simulink model "verify_Thermostat_Proportional_mdl"  (R2016b)
settings: Solver=ode45  StartTime=0.0  StopTime=100  MaxStep=1  RelTol=1e-3  EnableMultiTasking=on
libraries: simulink x1, carnot x1
settings Model: Creator=drhf  LastModifiedBy=drhf
settings DataIOCC: SaveFormat=Array  SignalLoggingSaveFormat=ModelDataLogs
settings OptimizationCC: ExpressionDepthLimit=2147483647  LifeSpan=inf
settings DebuggingCC: UnderspecifiedInitializationDetection=Classic  MergeDetectMultiDrivingBlocksExec=none  SolverPrmCheckMsg=warning  FcnCallInpInsideContextMsg=warning  StateNameClashWarn=warning  SFUnexpectedBacktrackingDiag=warning  SFNoUnconditionalDefaultTransitionDiag=warning  SFExecutionAtInitializationDiag=none
settings HardwareCC: ProdBitPerPointer=32  ProdBitPerSizeT=32  ProdBitPerPtrDiffT=32  ProdLargestAtomicFloat=None  ProdIntDivRoundTo=Undefined  ProdEndianess=Unspecified  ProdWordSize=32  ProdHWDeviceType=32-bit Generic
settings ModelReferenceCC: PropagateSignalLabelsOutOfModel=off
settings GRTTargetCC: TargetLangStandard=C89/C90 (ANSI)  GeneratePreprocessorConditionals=Disable all  CombineOutputUpdateFcns=off  GRTInterface=on
settings ConfigComp: CovMetricSettings=dw  CovHtmlReporting=on  CovSaveCumulativeToWorkspaceVar=on  CovSaveSingleToWorkspaceVar=on  CovExternalEMLEnable=off

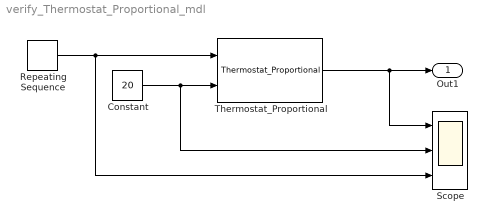
== system verify_Thermostat_Proportional_mdl ==
  Constant : Constant  Value=20
  Repeating Sequence : simulink/Sources/Repeating Sequence  rep_seq_t=[0 50 100]  rep_seq_y=[15 25 15]
  Scope : Scope  NumInputPorts=3
  Thermostat_Proportional : carnot/Control/Thermostat_Proportional  op=0.5  bl=0.2  p=4  ts=1
  Out1 : Outport  SampleTime=5
  wires:
  Thermostat_Proportional/1 -> Scope/1, Out1/1
  Repeating Sequence/1 -> Scope/3, Thermostat_Proportional/1
  Constant/1 -> Scope/2, Thermostat_Proportional/2
